simulink model "simulation"  (R2019a)
settings: Solver=VariableStepAuto  StartTime=0  StopTime=10  RelTol=1e-3
undefined symbols (not defined in the file or in its folder): gray
libraries: vrlib x4
settings Model: Creator=Mert Beser  LastModifiedBy=ecemi

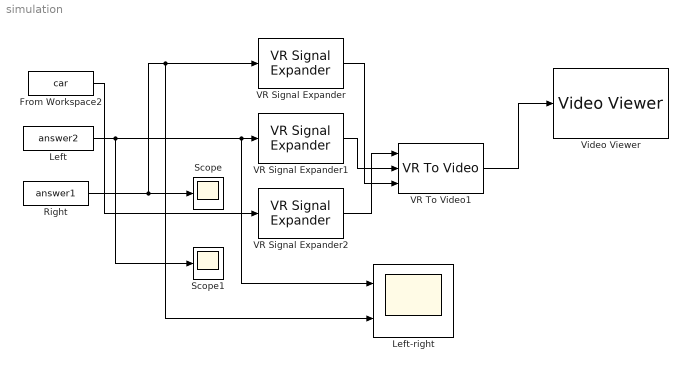
== system simulation ==
  From Workspace2 : FromWorkspace  VariableName=car  SampleTime=0
  Left : FromWorkspace  VariableName=answer2  SampleTime=0
  Left-right : Scope  NumInputPorts=2
  Right : FromWorkspace  VariableName=answer1  SampleTime=0
  Scope : Scope
  Scope1 : Scope
  VR Signal Expander : vrlib/VR Signal Expander  outwidth=4  outidx=[4]
      settings: SourceProductName=Simulink
  VR Signal Expander1 : vrlib/VR Signal Expander  outwidth=4  outidx=[4]
      settings: SourceProductName=Simulink
  VR Signal Expander2 : vrlib/VR Signal Expander  outwidth=3  outidx=[1]
      settings: SourceProductName=Simulink
  VR To Video1 : vrlib/VR To Video  InstantiateOnLoad=on  SampleTime=0.1  ViewEnable=on  RemoteChange=off  RemoteView=off  FieldsWritten=Box.translation.3.1.1.double#Eye_Left.rotation.4.1.1.double#Eye_Right.rotation.4.1.1.double  WorldFileName=C:\Users\ecemi\OneDrive\Masaüstü\simulation_environment.wrl  AutoView=off  VideoDimensions=[200 320]  AllowVariableSize=off
      settings: SourceProductName=Simulink  SourceProductBaseCode=SL
  Video Viewer : VideoViewer  colormapValue=gray(256)  FigPos=[1 678 1280 582.666666666667]
  wires:
  VR To Video1/1 -> Video Viewer/1
  Right/1 -> Left-right/2, VR Signal Expander/1, Scope/1
  Left/1 -> Scope1/1, Left-right/1, VR Signal Expander1/1
  From Workspace2/1 -> VR Signal Expander2/1
  VR Signal Expander2/1 -> VR To Video1/1
  VR Signal Expander1/1 -> VR To Video1/2
  VR Signal Expander/1 -> VR To Video1/3
